simulink model "ndof_realtime"  (R2024b)
settings: Solver=FixedStepAuto  StartTime=0.0  StopTime=10  FixedStep=min(T_state,Ts)  RelTol=1e-3
InitFcn:
  | init_fcn
StopFcn:
  | savedata
values from neighbouring files (symbols this model uses):
  ndof = 10    [init_fcn.m]    (also in ndofNE.m = ndofparams.ndof; ndofStateFunction.m = params(2))
  T_state = 0.01    [init_fcn.m]
  Ts = 0.01    [init_fcn.m]    (also in ndofStateFunction.m = params(1))
undefined symbols (not defined in the file or in its folder): DeviceSpecific, p, videoinput
libraries: sharedTrackingLibrary x1, imaqlib x1, simulink x1, visiongeotforms x1
settings Model: SimulationMode=accelerator  Creator=Haydar  LastModifiedBy=hayda
settings DataIOCC: SaveFormat=Array  SaveOutput=off  SignalLogging=off  DSMLogging=off

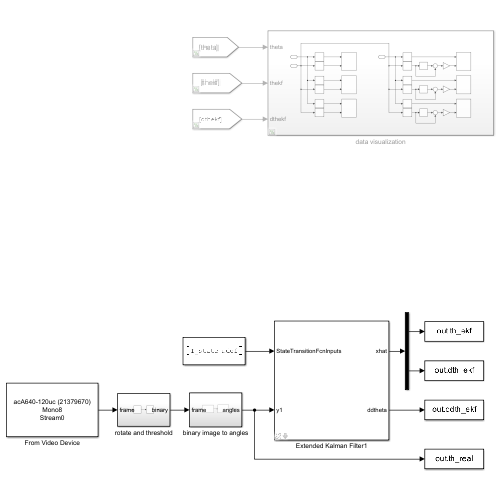
[thumbnail: Simulink's stored preview of the top-level diagram]
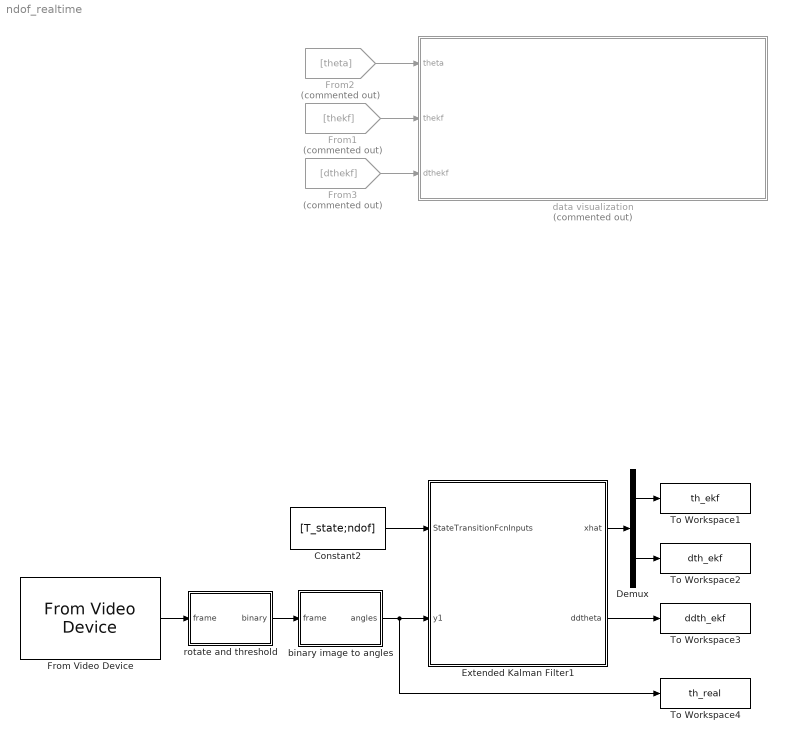
== system ndof_realtime ==
  Constant2 : Constant  Value=[T_state;ndof]
  Demux : Demux  Outputs=2
  Extended Kalman Filter1 : Subsystem  AncestorBlock=cstblocks/State Estimation/Extended Kalman Filter  mask(Extended Kalman Filter){StateTransitionFcn=ndofStateFunction, HasStateTransitionJacobianFcn=off, StateTransitionJacobianFcn=, HasAdditiveProcessNoise=Additive, ProcessNoise=0.02, HasTimeVaryingProcessNoise=off, HasStateTransitionFcnExtraArgument=1, InitialState=zeros(1,20), InitialStateCovariance=5, MeasurementFcn1=ndofMeasurementFunction, HasMeasurementJacobianFcn1=off, MeasurementJacobianFcn1=, HasMeasurementEnablePort1=off, HasAdditiveMeasurementNoise1=Additive, MeasurementNoise1=[20 25*ones(1,4) 30*ones(1,5)], HasTimeVaryingMeasurementNoise1=off, HasMeasurementFcnExtraArgument1=0, HasMeasurementWrapping1=off, MeasurementFcn2=myMeasurementFcn, HasMeasurementJacobianFcn2=off, MeasurementJacobianFcn2=, HasMeasurementEnablePort2=off, HasAdditiveMeasurementNoise2=Additive, MeasurementNoise2=1, HasTimeVaryingMeasurementNoise2=off, HasMeasurementFcnExtraArgument2=0, HasMeasurementWrapping2=off, MeasurementFcn3=myMeasurementFcn, HasMeasurementJacobianFcn3=off, MeasurementJacobianFcn3=, HasMeasurementEnablePort3=off, HasAdditiveMeasurementNoise3=Additive, MeasurementNoise3=1, HasTimeVaryingMeasurementNoise3=off, HasMeasurementFcnExtraArgument3=0, HasMeasurementWrapping3=off, MeasurementFcn4=myMeasurementFcn, HasMeasurementJacobianFcn4=off, MeasurementJacobianFcn4=, HasMeasurementEnablePort4=off, HasAdditiveMeasurementNoise4=Additive, MeasurementNoise4=1, HasTimeVaryingMeasurementNoise4=off, HasMeasurementFcnExtraArgument4=0, HasMeasurementWrapping4=off, MeasurementFcn5=myMeasurementFcn, HasMeasurementJacobianFcn5=off, MeasurementJacobianFcn5=, HasMeasurementEnablePort5=off, HasAdditiveMeasurementNoise5=Additive, MeasurementNoise5=1, HasTimeVaryingMeasurementNoise5=off, HasMeasurementFcnExtraArgument5=0, HasMeasurementWrapping5=off, EnableMultirate=on, StateTransitionFcnSampleTime=T_state, MeasurementFcn1SampleTime=Ts, MeasurementFcn2SampleTime=1, MeasurementFcn3SampleTime=1, MeasurementFcn4SampleTime=1, MeasurementFcn5SampleTime=1, UseCurrentEstimator=on, OutputStateCovariance=off, DataType=double, SampleTime=Ts, NumberOfMeasurements=1}
      mask prompts: HasStateTransitionJacobianFcn "shared_tracking:blocks:maskPromptEKFJacobian"; HasTimeVaryingProcessNoise "shared_tracking:blocks:maskPromptEKFUKFTimeVarying"; HasMeasurementJacobianFcn1 "shared_tracking:blocks:maskPromptEKFJacobian"; HasMeasurementEnablePort1 "shared_tracking:blocks:maskPromptEnablePort"; HasTimeVaryingMeasurementNoise1 "shared_tracking:blocks:maskPromptEKFUKFTimeVarying"; HasMeasurementWrapping1 "shared_tracking:blocks:maskPromptEKFUKFMeasurementWrapping"; HasMeasurementJacobianFcn2 "shared_tracking:blocks:maskPromptEKFJacobian"; HasMeasurementEnablePort2 "shared_tracking:blocks:maskPromptEnablePort"; HasTimeVaryingMeasurementNoise2 "shared_tracking:blocks:maskPromptEKFUKFTimeVarying"; HasMeasurementWrapping2 "shared_tracking:blocks:maskPromptEKFUKFMeasurementWrapping"; HasMeasurementJacobianFcn3 "shared_tracking:blocks:maskPromptEKFJacobian"; HasMeasurementEnablePort3 "shared_tracking:blocks:maskPromptEnablePort"; HasTimeVaryingMeasurementNoise3 "shared_tracking:blocks:maskPromptEKFUKFTimeVarying"; HasMeasurementWrapping3 "shared_tracking:blocks:maskPromptEKFUKFMeasurementWrapping"; HasMeasurementJacobianFcn4 "shared_tracking:blocks:maskPromptEKFJacobian"; HasMeasurementEnablePort4 "shared_tracking:blocks:maskPromptEnablePort"; HasTimeVaryingMeasurementNoise4 "shared_tracking:blocks:maskPromptEKFUKFTimeVarying"; HasMeasurementWrapping4 "shared_tracking:blocks:maskPromptEKFUKFMeasurementWrapping"; HasMeasurementJacobianFcn5 "shared_tracking:blocks:maskPromptEKFJacobian"; HasMeasurementEnablePort5 "shared_tracking:blocks:maskPromptEnablePort"; HasTimeVaryingMeasurementNoise5 "shared_tracking:blocks:maskPromptEKFUKFTimeVarying"; HasMeasurementWrapping5 "shared_tracking:blocks:maskPromptEKFUKFMeasurementWrapping"; EnableMultirate "shared_tracking:blocks:maskPromptEnableMultirate"; StateTransitionFcnSampleTime "shared_tracking:blocks:maskPromptStateTransition"; MeasurementFcn1SampleTime "shared_tracking:blocks:maskPromptMeasurement1"; MeasurementFcn2SampleTime "shared_tracking:blocks:maskPromptMeasurement2"; MeasurementFcn3SampleTime "shared_tracking:blocks:maskPromptMeasurement3"; MeasurementFcn4SampleTime "shared_tracking:blocks:maskPromptMeasurement4"; MeasurementFcn5SampleTime "shared_tracking:blocks:maskPromptMeasurement5"; UseCurrentEstimator "shared_tracking:blocks:maskPromptUseCurrentEstimator"; OutputStateCovariance "shared_tracking:blocks:maskPromptOutputStateCovariance"; DataType "shared_tracking:blocks:maskPromptDataType"; SampleTime "shared_tracking:blocks:maskPromptSampleTime"
      mask help: shared_tracking:blocks:maskPromptEKFDescription
      mask init:
      | matlabshared.tracking.internal.blocks.maskInitializationScriptEKF
      settings: LibrarySourceBlock=cstblocks/State Estimation/Extended Kalman Filter
      mask Help: eval('matlabshared.tracking.internal.blocks.controlIdentLaunchDocPage(''EKF'')')
      mask Callback HasStateTransitionJacobianFcn: matlabshared.tracking.internal.blocks.dialogCallbacksEKFUKFPF(gcbh(),'checkBoxHasJacobianFcn','StateTransition');
      mask TypeOptions HasAdditiveProcessNoise: shared_tracking:blocks:maskPromptEKFUKFAdditiveNoise | shared_tracking:blocks:maskPromptEKFUKFNonAdditiveNoise
      mask Callback HasTimeVaryingProcessNoise: matlabshared.tracking.internal.blocks.dialogCallbacksEKFUKFPF(gcbh,'checkboxIsCovarianceTimeVarying','HasTimeVaryingProcessNoise','ProcessNoise')
      mask Callback HasMeasurementJacobianFcn1: matlabshared.tracking.internal.blocks.dialogCallbacksEKFUKFPF(gcbh(),'checkBoxHasJacobianFcn','Measurement','1');
      mask TypeOptions HasAdditiveMeasurementNoise1: shared_tracking:blocks:maskPromptEKFUKFAdditiveNoise | shared_tracking:blocks:maskPromptEKFUKFNonAdditiveNoise
      mask Callback HasTimeVaryingMeasurementNoise1: matlabshared.tracking.internal.blocks.dialogCallbacksEKFUKFPF(gcbh,'checkboxIsCovarianceTimeVarying','HasTimeVaryingMeasurementNoise1','MeasurementNoise1')
      mask Callback HasMeasurementJacobianFcn2: matlabshared.tracking.internal.blocks.dialogCallbacksEKFUKFPF(gcbh(),'checkBoxHasJacobianFcn','Measurement','2');
      mask TypeOptions HasAdditiveMeasurementNoise2: shared_tracking:blocks:maskPromptEKFUKFAdditiveNoise | shared_tracking:blocks:maskPromptEKFUKFNonAdditiveNoise
      mask Callback HasTimeVaryingMeasurementNoise2: matlabshared.tracking.internal.blocks.dialogCallbacksEKFUKFPF(gcbh,'checkboxIsCovarianceTimeVarying','HasTimeVaryingMeasurementNoise2','MeasurementNoise2')
      mask Callback HasMeasurementJacobianFcn3: matlabshared.tracking.internal.blocks.dialogCallbacksEKFUKFPF(gcbh(),'checkBoxHasJacobianFcn','Measurement','3');
      mask TypeOptions HasAdditiveMeasurementNoise3: shared_tracking:blocks:maskPromptEKFUKFAdditiveNoise | shared_tracking:blocks:maskPromptEKFUKFNonAdditiveNoise
      mask Callback HasTimeVaryingMeasurementNoise3: matlabshared.tracking.internal.blocks.dialogCallbacksEKFUKFPF(gcbh,'checkboxIsCovarianceTimeVarying','HasTimeVaryingMeasurementNoise3','MeasurementNoise3')
      mask Callback HasMeasurementJacobianFcn4: matlabshared.tracking.internal.blocks.dialogCallbacksEKFUKFPF(gcbh(),'checkBoxHasJacobianFcn','Measurement','4');
      mask TypeOptions HasAdditiveMeasurementNoise4: shared_tracking:blocks:maskPromptEKFUKFAdditiveNoise | shared_tracking:blocks:maskPromptEKFUKFNonAdditiveNoise
      mask Callback HasTimeVaryingMeasurementNoise4: matlabshared.tracking.internal.blocks.dialogCallbacksEKFUKFPF(gcbh,'checkboxIsCovarianceTimeVarying','HasTimeVaryingMeasurementNoise4','MeasurementNoise4')
      mask Callback HasMeasurementJacobianFcn5: matlabshared.tracking.internal.blocks.dialogCallbacksEKFUKFPF(gcbh(),'checkBoxHasJacobianFcn','Measurement','5');
      mask TypeOptions HasAdditiveMeasurementNoise5: shared_tracking:blocks:maskPromptEKFUKFAdditiveNoise | shared_tracking:blocks:maskPromptEKFUKFNonAdditiveNoise
      mask Callback HasTimeVaryingMeasurementNoise5: matlabshared.tracking.internal.blocks.dialogCallbacksEKFUKFPF(gcbh,'checkboxIsCovarianceTimeVarying','HasTimeVaryingMeasurementNoise5','MeasurementNoise5')
      mask Callback EnableMultirate: matlabshared.tracking.internal.blocks.dialogCallbacksEKFUKFPF(gcbh,'checkBoxHasMultirate')
      mask TypeOptions DataType: shared_tracking:blocks:maskPromptDouble | shared_tracking:blocks:maskPromptSingle
      mask Callback NumberOfMeasurements: matlabshared.tracking.internal.blocks.dialogCallbacksEKFUKFPF(gcbh,'editboxNumberOfMeasurements','MeasurementFcn');
      mask DialogControl DescGroupVar Prompt: shared_tracking:blocks:maskPromptEKFTitle
      mask DialogControl TabSystemModel Prompt: shared_tracking:blocks:maskPromptSystemModel
      mask DialogControl GroupStateTransition Prompt: shared_tracking:blocks:maskPromptStateTransition
      mask DialogControl StateTransitionFunctionText Prompt: shared_tracking:blocks:maskPromptFunction
      mask DialogControl HasStateTransitionJacobianFcn Prompt: Jacobian
      mask DialogControl ProcessNoiseText Prompt: shared_tracking:blocks:maskPromptEKFUKFProcessNoise
      mask DialogControl ProcessNoiseCovarianceText Prompt: shared_tracking:blocks:maskPromptCovariance
      mask DialogControl HasTimeVaryingProcessNoise Prompt: Time-varying
      mask DialogControl InitializationContainer Prompt: shared_tracking:blocks:maskPromptInitialization
      mask DialogControl InitialStateText Prompt: shared_tracking:blocks:maskPromptEKFUKFInitialState
      mask DialogControl InitialCovarianceText Prompt: shared_tracking:blocks:maskPromptEKFUKFInitialCovariance
      mask DialogControl GroupMeasurement1 Prompt: shared_tracking:blocks:maskPromptMeasurement1
      mask DialogControl MeasurementFunction1Text Prompt: shared_tracking:blocks:maskPromptFunction
      mask DialogControl HasMeasurementJacobianFcn1 Prompt: Jacobian
      mask DialogControl HasMeasurementEnablePort1 Prompt: Add Enable port
      mask DialogControl MeasurementNoiseText1 Prompt: shared_tracking:blocks:maskPromptEKFUKFMeasurementNoise
      mask DialogControl MeasurementNoiseCovarianceText1 Prompt: shared_tracking:blocks:maskPromptCovariance
      mask DialogControl HasTimeVaryingMeasurementNoise1 Prompt: Time-varying
      mask DialogControl HasMeasurementWrapping1 Prompt: Enable measurement wrapping
      mask DialogControl GroupMeasurement2 Prompt: shared_tracking:blocks:maskPromptMeasurement2
      mask DialogControl MeasurementFunction2Text Prompt: shared_tracking:blocks:maskPromptFunction
      mask DialogControl HasMeasurementJacobianFcn2 Prompt: Jacobian
      mask DialogControl HasMeasurementEnablePort2 Prompt: Add Enable port
      mask DialogControl MeasurementNoiseText2 Prompt: shared_tracking:blocks:maskPromptEKFUKFMeasurementNoise
      mask DialogControl MeasurementNoiseCovarianceText2 Prompt: shared_tracking:blocks:maskPromptCovariance
      mask DialogControl HasTimeVaryingMeasurementNoise2 Prompt: Time-varying
      mask DialogControl HasMeasurementWrapping2 Prompt: Enable measurement wrapping
      mask DialogControl GroupMeasurement3 Prompt: shared_tracking:blocks:maskPromptMeasurement3
      mask DialogControl MeasurementFunction3Text Prompt: shared_tracking:blocks:maskPromptFunction
      mask DialogControl HasMeasurementJacobianFcn3 Prompt: Jacobian
      mask DialogControl HasMeasurementEnablePort3 Prompt: Add Enable port
      mask DialogControl MeasurementNoiseText3 Prompt: shared_tracking:blocks:maskPromptEKFUKFMeasurementNoise
      mask DialogControl MeasurementNoiseCovarianceText3 Prompt: shared_tracking:blocks:maskPromptCovariance
      mask DialogControl HasTimeVaryingMeasurementNoise3 Prompt: Time-varying
      mask DialogControl HasMeasurementWrapping3 Prompt: Enable measurement wrapping
      mask DialogControl GroupMeasurement4 Prompt: shared_tracking:blocks:maskPromptMeasurement4
      mask DialogControl MeasurementFunction4Text Prompt: shared_tracking:blocks:maskPromptFunction
      mask DialogControl HasMeasurementJacobianFcn4 Prompt: Jacobian
      mask DialogControl HasMeasurementEnablePort4 Prompt: Add Enable port
      mask DialogControl MeasurementNoiseText4 Prompt: shared_tracking:blocks:maskPromptEKFUKFMeasurementNoise
      mask DialogControl MeasurementNoiseCovarianceText4 Prompt: shared_tracking:blocks:maskPromptCovariance
      mask DialogControl HasTimeVaryingMeasurementNoise4 Prompt: Time-varying
      mask DialogControl HasMeasurementWrapping4 Prompt: Enable measurement wrapping
      mask DialogControl GroupMeasurement5 Prompt: shared_tracking:blocks:maskPromptMeasurement5
      mask DialogControl MeasurementFunction5Text Prompt: shared_tracking:blocks:maskPromptFunction
      mask DialogControl HasMeasurementJacobianFcn5 Prompt: Jacobian
      mask DialogControl HasMeasurementEnablePort5 Prompt: Add Enable port
      mask DialogControl MeasurementNoiseText5 Prompt: shared_tracking:blocks:maskPromptEKFUKFMeasurementNoise
      mask DialogControl MeasurementNoiseCovarianceText5 Prompt: shared_tracking:blocks:maskPromptCovariance
      mask DialogControl HasTimeVaryingMeasurementNoise5 Prompt: Time-varying
      mask DialogControl HasMeasurementWrapping5 Prompt: Enable measurement wrapping
      mask DialogControl AddMeasurement Prompt: shared_tracking:blocks:maskPromptAddMeasurement
      mask DialogControl AddMeasurement Callback: matlabshared.tracking.internal.blocks.dialogCallbacksEKFUKFPF(gcbh,'buttonAddMeasurement','MeasurementFcn');
      mask DialogControl RemoveMeasurement Prompt: shared_tracking:blocks:maskPromptRemoveMeasurement
      mask DialogControl RemoveMeasurement Callback: matlabshared.tracking.internal.blocks.dialogCallbacksEKFUKFPF(gcbh,'buttonRemoveMeasurement','MeasurementFcn');
      mask DialogControl TabMultirate Prompt: shared_tracking:blocks:maskPromptEKFUKFMultirate
      mask DialogControl GroupMultirate Prompt: shared_tracking:blocks:maskPromptEKFUKFMultirate
      mask DialogControl EnableMultirate Prompt: Enable multirate operation
      mask DialogControl GroupMultirateSampleTimes Prompt: shared_tracking:blocks:maskPromptSampleTimeNoInheritance
      mask DialogControl StateTransitionFcnSampleTime Prompt: State Transition
      mask DialogControl MeasurementFcn1SampleTime Prompt: Measurement 1
      mask DialogControl MeasurementFcn2SampleTime Prompt: Measurement 2
      mask DialogControl MeasurementFcn3SampleTime Prompt: Measurement 3
      mask DialogControl MeasurementFcn4SampleTime Prompt: Measurement 4
      mask DialogControl MeasurementFcn5SampleTime Prompt: Measurement 5
      mask DialogControl ContainerSettings Prompt: shared_tracking:blocks:maskPromptEKFUKFSettings
      mask DialogControl UseCurrentEstimator Prompt: Use the current measurements to improve state estimates
      mask DialogControl OutputStateCovariance Prompt: Output state estimation error covariance
      mask DialogControl DataType Prompt: Data type:
      mask DialogControl SampleTime Prompt: Sample time:
  From Video Device : imaqlib/From Video Device  DeviceMenu=(none)  Device=gentl 1 (acA640-120uc (21379670))  ObjConstructor=videoinput('gentl', 1)  VideoFormatMenu=(none)  VideoFormat=Mono8  VideoSource=Stream0  ROIPosition=[0 0 492 658]  EnableHWTrigger=off  TriggerConfiguration=DeviceSpecific/DeviceSpecific  SampleTime=0.01  OutputPortsMode=One multidimensional signal  DataType=uint8  CanDoHWTrigger=yes  ReturnedColorSpace=grayscale  BlockHandle=156.0001  ROIWidth=658  ROIHeight=492  ROIColumn=0  ROIRow=0  EngXMLPath=C:\Program Files\MATLAB\R2024b\toolbox\imaq\imaq\private  DevXMLPath=C:\ProgramData\MATLAB\SupportPackages\R2024b\toolbox\imaq\supportpackages\gentl\adaptor\win64  EngLibPath=C:\Program Files\MATLAB\R2024b\toolbox\imaq\imaqblks\imaqmex\win64  ColorSpace=grayscale  BayerSensorAlignment=grbg  ImaqMode=off
  From1 : From  Commented=on  GotoTag=thekf
  From2 : From  Commented=on  GotoTag=theta
  From3 : From  Commented=on  GotoTag=dthekf
  To Workspace1 : ToWorkspace  VariableName=th_ekf  SampleTime=0.01
  To Workspace2 : ToWorkspace  VariableName=dth_ekf  SampleTime=0.01
  To Workspace3 : ToWorkspace  VariableName=ddth_ekf  SampleTime=0.01
  To Workspace4 : ToWorkspace  VariableName=th_real  SampleTime=0.01
  binary image to angles : Subsystem
  data visualization : Subsystem  Commented=on
  rotate and threshold : Subsystem
  wires:
  Constant2/1 -> Extended Kalman Filter1/1(StateTransitionFcnInputs)
  Extended Kalman Filter1/1(xhat) -> Demux/1
  Demux/2 -> To Workspace2/1
  Demux/1 -> To Workspace1/1
  Extended Kalman Filter1/2(ddtheta) -> To Workspace3/1
  From1/1 -> data visualization/2(thekf)
  From2/1 -> data visualization/1(theta)
  From3/1 -> data visualization/3(dthekf)
  binary image to angles/1(angles) -> To Workspace4/1, Extended Kalman Filter1/2(y1)
  From Video Device/1 -> rotate and threshold/1(frame)
  rotate and threshold/1(binary) -> binary image to angles/1(frame)

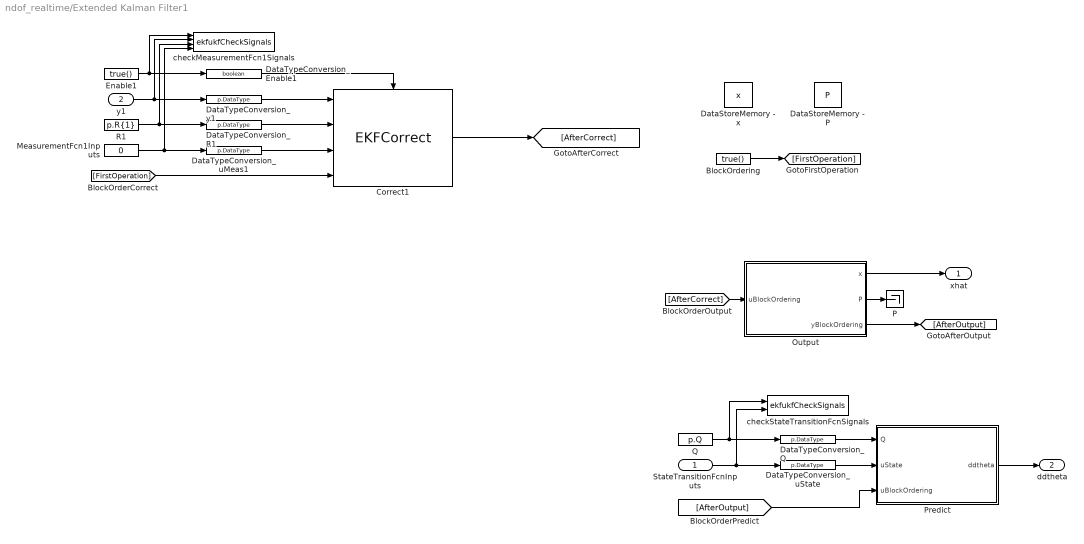
== system ndof_realtime/Extended Kalman Filter1 ==
  StateTransitionFcnInputs : Inport
  y1 : Inport  Port=2
  BlockOrdering : Constant  Value=true()  OutDataTypeStr=boolean
  Correct1 : sharedTrackingLibrary/Extras/EKFCorrect  ProcessedMaskData=p
  DataStoreMemory - P : DataStoreMemory  DataStoreName=P  InitialValue=p.InitialCovariance  ShowAdditionalParam=off  OutDataTypeStr=p.DataType
  DataStoreMemory - x : DataStoreMemory  DataStoreName=x  InitialValue=p.InitialState  ShowAdditionalParam=off  OutDataTypeStr=p.DataType
  DataTypeConversion_Enable1 : DataTypeConversion  OutDataTypeStr=boolean  SaturateOnIntegerOverflow=off  RndMeth=Floor
  DataTypeConversion_Q : DataTypeConversion  OutDataTypeStr=p.DataType  SaturateOnIntegerOverflow=off  RndMeth=Floor
  DataTypeConversion_R1 : DataTypeConversion  OutDataTypeStr=p.DataType  SaturateOnIntegerOverflow=off  RndMeth=Floor
  DataTypeConversion_uMeas1 : DataTypeConversion  OutDataTypeStr=p.DataType  SaturateOnIntegerOverflow=off  RndMeth=Floor
  DataTypeConversion_uState : DataTypeConversion  OutDataTypeStr=p.DataType  SaturateOnIntegerOverflow=off  RndMeth=Floor
  DataTypeConversion_y1 : DataTypeConversion  OutDataTypeStr=p.DataType  SaturateOnIntegerOverflow=off  RndMeth=Floor
  Enable1 : Constant  Value=true()  SampleTime=p.SampleTimes.MeasurementFcn(1)
  MeasurementFcn1Inputs : Constant  Value=0  OutDataTypeStr=p.DataType  SampleTime=p.SampleTimes.MeasurementFcn(1)
  Output : Subsystem  TreatAsAtomicUnit=on  SystemSampleTime=p.SampleTimes.Output
  P : Terminator
  Predict : Subsystem  TreatAsAtomicUnit=on  SystemSampleTime=p.SampleTimes.StateTransitionFcn  mask(EKFPredict){ProcessedMaskData=p}
      mask init:
      | if strcmp(get_param(bdroot,'SimulationStatus'),'stopped')
      |     pS = [];
      |     SampleTime = [];
      |     DataType = [];
      |     SLFcnsToRegister = {};
      | else
      |     [pS,SampleTime] = ...
      |         matlabshared.tracking.internal.blocks.maskInitializationFcnEKFPredictor(ProcessedMaskData);
      |     [DataType,SLFcnsToRegister] = ...
      |         matlabshared.tracking.internal.blocks.maskInitializationFcnRegisterSLFcn(ProcessedMaskData, pS);
      | end
  Q : Constant  Value=p.Q  SampleTime=p.SampleTimes.StateTransitionFcn
  R1 : Constant  Value=p.R{1}  SampleTime=p.SampleTimes.MeasurementFcn(1)
  checkMeasurementFcn1Signals : S-Function  FunctionName=ekfukfCheckSignals  Parameters=signalCheck.BlockPath, signalCheck.MeasurementFcn{1}.PortNames, signalCheck.MeasurementFcn{1}.SampleTime, signalCheck.DataType, signalCheck.MeasurementFcn{1}.PortDimensions, 1, signalCheck.MeasurementFcn{1}.HasAdditiveNoise  SFunctionDeploymentMode=off  EnableBusSupport=off
  checkStateTransitionFcnSignals : S-Function  FunctionName=ekfukfCheckSignals  Parameters=signalCheck.BlockPath, signalCheck.StateTransitionFcn.PortNames, signalCheck.StateTransitionFcn.SampleTime, signalCheck.DataType, signalCheck.StateTransitionFcn.PortDimensions, 0, signalCheck.StateTransitionFcn.HasAdditiveNoise  SFunctionDeploymentMode=off  EnableBusSupport=off
  xhat : Outport  VectorParamsAs1DForOutWhenUnconnected=off
  ddtheta : Outport  Port=2
  wires:
  Predict/1(ddtheta) -> ddtheta/1
  y1/1 -> checkMeasurementFcn1Signals/2, DataTypeConversion_y1/1
  R1/1 -> checkMeasurementFcn1Signals/3, DataTypeConversion_R1/1
  Q/1 -> checkStateTransitionFcnSignals/1, DataTypeConversion_Q/1
  DataTypeConversion_Q/1 -> Predict/1(Q)
  Enable1/1 -> checkMeasurementFcn1Signals/1, DataTypeConversion_Enable1/1
  DataTypeConversion_Enable1/1 -> Correct1/Enable
  Output/2(P) -> P/1
  Output/1(x) -> xhat/1
  StateTransitionFcnInputs/1 -> checkStateTransitionFcnSignals/2, DataTypeConversion_uState/1
  DataTypeConversion_uState/1 -> Predict/2(uState)
  DataTypeConversion_y1/1 -> Correct1/1
  MeasurementFcn1Inputs/1 -> checkMeasurementFcn1Signals/4, DataTypeConversion_uMeas1/1
  DataTypeConversion_R1/1 -> Correct1/2
  DataTypeConversion_uMeas1/1 -> Correct1/3
  BlockOrdering/1 -> [FirstOperation]
  [FirstOperation] -> Correct1/4
  [AfterCorrect] -> Output/1(uBlockOrdering)
  Output/3(yBlockOrdering) -> [AfterOutput]
  Correct1/1 -> [AfterCorrect]
  [AfterOutput] -> Predict/3(uBlockOrdering)

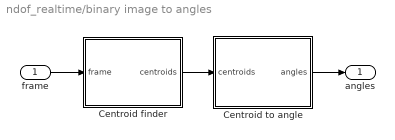
== system ndof_realtime/binary image to angles ==
  frame : Inport
  Centroid finder : MATLAB Function  TreatAsAtomicUnit=on
  Centroid to angle : MATLAB Function  TreatAsAtomicUnit=on
  angles : Outport
  wires:
  Centroid to angle/1(angles) -> angles/1
  Centroid finder/1(centroids) -> Centroid to angle/1(centroids)
  frame/1 -> Centroid finder/1(frame)

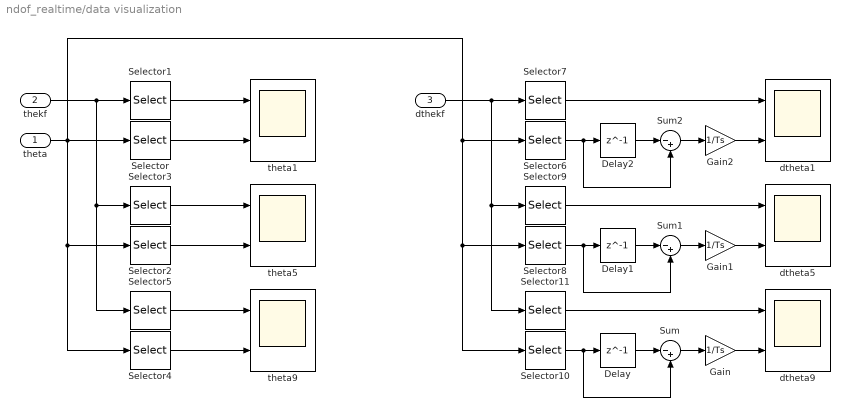
== system ndof_realtime/data visualization ==
  theta : Inport
  thekf : Inport  Port=2
  dthekf : Inport  Port=3
  Delay : Delay  DelayLength=1  SampleTime=Ts
  Delay1 : Delay  DelayLength=1  SampleTime=Ts
  Delay2 : Delay  DelayLength=1  SampleTime=Ts
  Gain : Gain  Gain=1/Ts
  Gain1 : Gain  Gain=1/Ts
  Gain2 : Gain  Gain=1/Ts
  Selector{,1,6..7} (4 alike) : Selector  InputPortWidth=10  IndexOptions=Index vector (dialog)  Indices=1  OutputSizes=1
  Selector{4..5,10..11} (4 alike) : Selector  InputPortWidth=10  IndexOptions=Index vector (dialog)  Indices=9  OutputSizes=1
  Selector{2..3,8..9} (4 alike) : Selector  InputPortWidth=10  IndexOptions=Index vector (dialog)  Indices=5  OutputSizes=1
  Sum : Sum  Inputs=|-+
  Sum1 : Sum  Inputs=|-+
  Sum2 : Sum  Inputs=|-+
  dtheta1 : Scope  NumInputPorts=2
  dtheta5 : Scope  NumInputPorts=2
  dtheta9 : Scope  NumInputPorts=2
  theta1 : Scope  NumInputPorts=2
  theta5 : Scope  NumInputPorts=2
  theta9 : Scope  NumInputPorts=2
  wires:
  Selector3/1 -> theta5/1
  dthekf/1 -> Selector7/1, Selector11/1, Selector9/1
  Selector4/1 -> theta9/2
  Selector2/1 -> theta5/2
  Selector10/1 -> Sum/2, Delay/1
  theta/1 -> Selector/1, Selector6/1, Selector10/1, Selector8/1, Selector4/1, Selector2/1
  Gain/1 -> dtheta9/2
  Selector9/1 -> dtheta5/1
  thekf/1 -> Selector1/1, Selector5/1, Selector3/1
  Selector5/1 -> theta9/1
  Selector/1 -> theta1/2
  Selector7/1 -> dtheta1/1
  Selector11/1 -> dtheta9/1
  Selector1/1 -> theta1/1
  Delay/1 -> Sum/1
  Sum/1 -> Gain/1
  Selector8/1 -> Sum1/2, Delay1/1
  Delay1/1 -> Sum1/1
  Sum1/1 -> Gain1/1
  Gain1/1 -> dtheta5/2
  Gain2/1 -> dtheta1/2
  Selector6/1 -> Sum2/2, Delay2/1
  Delay2/1 -> Sum2/1
  Sum2/1 -> Gain2/1

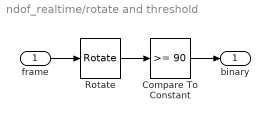
== system ndof_realtime/rotate and threshold ==
  frame : Inport
  Compare To Constant : simulink/Logic and Bit Operations/Compare To Constant  relop=>=  const=90  OutDataTypeStr=boolean
  Rotate : visiongeotforms/Rotate  outSizeR=Expanded to fit rotated input image  src_angle=Specify via dialog  unit_angle=Degrees  angle=-pi/2  maxAngle=pi  dispImage=Top-left corner  method=Table lookup  fillVal=0  interpMethod=Bilinear  roundingMode=Round  overflowMode=on  prodOutputMode=Binary point scaling  prodOutputWordLength=32  prodOutputFracLength=10
  binary : Outport
  wires:
  Rotate/1 -> Compare To Constant/1
  Compare To Constant/1 -> binary/1
  frame/1 -> Rotate/1

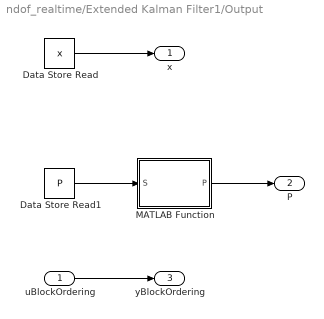
== system ndof_realtime/Extended Kalman Filter1/Output ==
  uBlockOrdering : Inport
  Data Store Read : DataStoreRead  DataStoreName=x  IndexOptions=Index vector (dialog)  Indices=1  OutputSizes=1
  Data Store Read1 : DataStoreRead  DataStoreName=P  IndexOptions=Index vector (dialog)  Indices=1  OutputSizes=1
  MATLAB Function : MATLAB Function  TreatAsAtomicUnit=on
  x : Outport  VectorParamsAs1DForOutWhenUnconnected=off
  P : Outport  Port=2  VectorParamsAs1DForOutWhenUnconnected=off
  yBlockOrdering : Outport  Port=3  VectorParamsAs1DForOutWhenUnconnected=off
  wires:
  Data Store Read/1 -> x/1
  Data Store Read1/1 -> MATLAB Function/1(S)
  uBlockOrdering/1 -> yBlockOrdering/1
  MATLAB Function/1(P) -> P/1

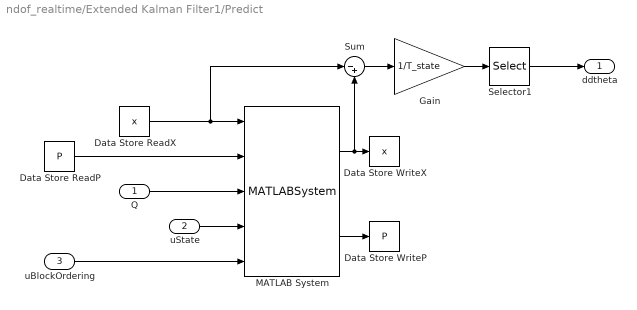
== system ndof_realtime/Extended Kalman Filter1/Predict ==
  Q : Inport  SampleTime=SampleTime
  uState : Inport  Port=2  SampleTime=SampleTime
  uBlockOrdering : Inport  Port=3  SampleTime=SampleTime
  Data Store WriteP : DataStoreWrite  DataStoreName=P  IndexOptions=Index vector (dialog)  Indices=1  OutputSizes=1
  Data Store WriteX : DataStoreWrite  DataStoreName=x  IndexOptions=Index vector (dialog)  Indices=1  OutputSizes=1
  Data Store ReadP : DataStoreRead  DataStoreName=P  IndexOptions=Index vector (dialog)  Indices=1  OutputSizes=1
  Data Store ReadX : DataStoreRead  DataStoreName=x  IndexOptions=Index vector (dialog)  Indices=1  OutputSizes=1
  Gain : Gain  Gain=1/T_state
  MATLAB System : MATLABSystem  System=matlabshared.tracking.internal.blocks.ekfPredictFcn  DlgParamStruct=pS  SLFcn=SLFcnsToRegister  DataType=DataType  SimulateUsing=Code generation
      mask Type: matlabshared.tracking.internal.blocks.ekfPredictFcn
      mask Display:
      | disp('ekfPredictFcn');
      | port_label('input',1,'x');
      | port_label('input',2,'P');
      | port_label('input',3,'Q');
      | port_label('input',4,'uState');
      | port_label('input',5,'~');
      | port_label('output',1,'xNew');
      | port_label('output',2,'P');
  Selector1 : Selector  InputPortWidth=20  IndexOptions=Index vector (dialog)  Indices=11:20  OutputSizes=1
  Sum : Sum  Inputs=|-+
  ddtheta : Outport
  wires:
  Selector1/1 -> ddtheta/1
  Gain/1 -> Selector1/1
  Sum/1 -> Gain/1
  Data Store ReadP/1 -> MATLAB System/2
  MATLAB System/2 -> Data Store WriteP/1
  Q/1 -> MATLAB System/3
  MATLAB System/1 -> Data Store WriteX/1, Sum/2
  Data Store ReadX/1 -> MATLAB System/1, Sum/1
  uState/1 -> MATLAB System/4
  uBlockOrdering/1 -> MATLAB System/5

== matlab function ndof_realtime/binary image to angles/Centroid to angle ==
  data: centroids input; angles output
function angles= fcn(centroids)
N = length(centroids);
angles = zeros(N-1,1);
for i = 1:N-1
    if i == 1
        a = centroids(i, :) - [0 1];
        b = centroids(i, :);
        c = centroids(i+1,:);

        u1 = [b(1) - a(1); b(2) - a(2); 0];
        u2 = [c(1) - b(1); c(2) - b(2); 0];

        do = u1(1)*u2(1) + u1(2)*u2(2);
        cr = u1(1)*u2(2) - u1(2)*u2(1);

        angles(i) = -atan2(cr, do);
    else
        a = centroids(i-1,:);
        b = centroids(i, :);
        c = centroids(i+1,:);

        u1 = [b(1) - a(1); b(2) - a(2); 0];
        u2 = [c(1) - b(1); c(2) - b(2); 0];

        do = u1(1)*u2(1) + u1(2)*u2(2);
        cr = u1(1)*u2(2) - u1(2)*u2(1);

        angles(i) = -atan2(cr, do);
    end
end

== matlab function ndof_realtime/Extended Kalman Filter1/Output/MATLAB Function ==
  data: S input; P output
function P = fcn(S)
    
    % Get back Covariance from Square-root Covariance
    P = S*S';
    
end

== matlab function ndof_realtime/binary image to angles/Centroid finder ==
  data: frame input; centroids output
function centroids = fcn(frame)
rp = regionprops(frame, 'Centroid');
N = 11;
centroids = zeros(N,2);

c = zeros(N,2);
for i = 1:N
    c(i,:) = rp(i).Centroid;
end


[~, idx] = sort(c(:,2), 1);
centroids(:,:) = c(idx, :);
